simulink subsystem "PROGRAM_COUNTER_06_SS"  (R2022a)
settings: Solver=VariableStepAuto  StartTime=0.0  StopTime=10.0  RelTol=1e-3
libraries: hdlBasic x1928, hlsBasic x1
(part 1 of 12)
settings Model: Creator=sebas  LastModifiedBy=sebas

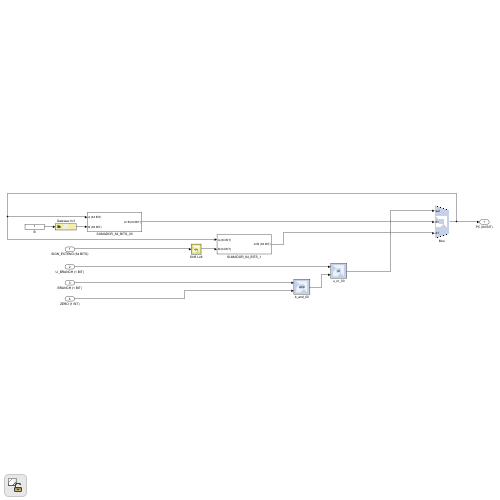
[thumbnail: Simulink's stored preview of the top-level diagram]
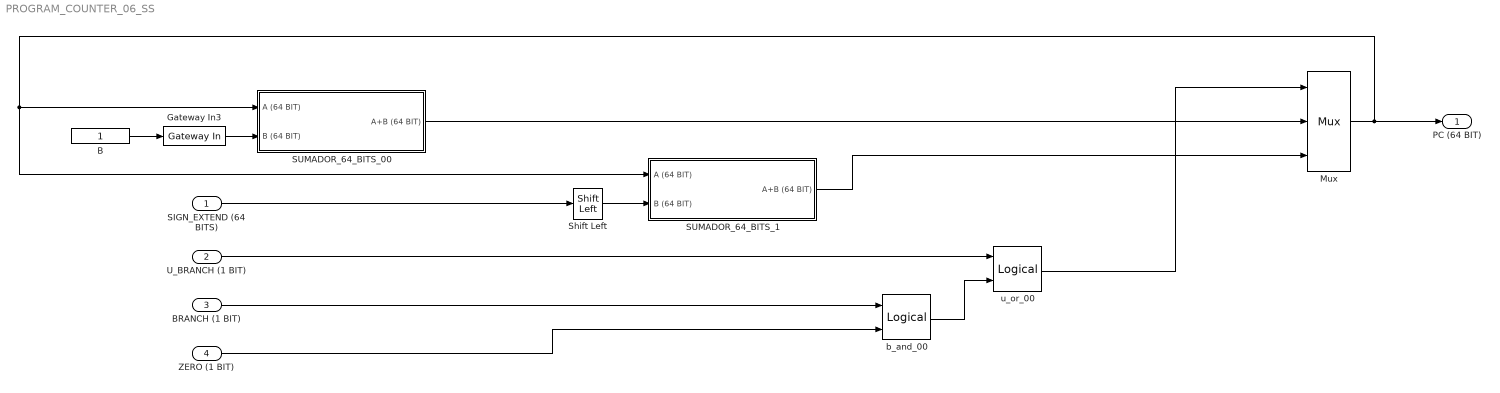
== system PROGRAM_COUNTER_06_SS ==
  SIGN_EXTEND (64 BITS) : Inport
  U_BRANCH (1 BIT) : Inport  Port=2
  BRANCH (1 BIT) : Inport  Port=3
  ZERO (1 BIT) : Inport  Port=4
  B : Constant
  Gateway In3 : hdlBasic/Gateway In  gui_display_data_type=Fixed-point  arith_type=Unsigned  n_bits=1  bin_pt=0  preci_type=Single  exp_width=8  frac_width=24  rows=1  columns=1  quantization="Round  (unbiased: +/- Inf)"  overflow=Saturate  period=1  UseAsADC=off  ADCChannel='1'  interface=None  automatic_assignment=on  address_offset=hex2dec('00')  intf_name=''  intf_description=''  default_value=0  timing_constraint=None  locs_specified=off  LOCs={}  io_standard={}  inherit_from_input=off  hdl_port=on  XmcBlockStatus=1  maskContainerNames=group4  block_type=gatewayin  block_config=sysgen:gateway_in_config  block_width_w=590  block_height_w=620  block_width=640  block_height=850
  Mux : hdlBasic/Mux  inputs=2  en=off  latency=0  precision=Full  arith_type=Unsigned  n_bits=16  bin_pt=14  quantization=Truncate  overflow=Wrap  XmcBlockStatus=1  maskContainerNames=tabcontainer1  block_type=mux  block_config=sysgen:Mux_config
  SUMADOR_64_BITS_00 : Subsystem
  SUMADOR_64_BITS_1 : Subsystem
  Shift Left : hlsBasic/Shift Left  ShiftAmount=2
  b_and_00 : hdlBasic/Logical  logical_function=AND  inputs=2  en=off  latency=0  precision=Full  arith_type=Unsigned  n_bits=16  bin_pt=0  align_bp=on  overflow=[]  quantization=[]  XmcBlockStatus=1  maskContainerNames=tabcontainer1  block_type=logical  block_config=sysgen:Logical_config
  u_or_00 : hdlBasic/Logical  logical_function=OR  inputs=2  en=off  latency=0  precision=Full  arith_type=Unsigned  n_bits=16  bin_pt=0  align_bp=on  overflow=[]  quantization=[]  XmcBlockStatus=1  maskContainerNames=tabcontainer1  block_type=logical  block_config=sysgen:Logical_config
  PC (64 BIT) : Outport
  wires:
  ZERO (1 BIT)/1 -> b_and_00/2
  SUMADOR_64_BITS_1/1(A+B (64 BIT)) -> Mux/3
  SUMADOR_64_BITS_00/1(A+B (64 BIT)) -> Mux/2
  u_or_00/1 -> Mux/1
  Gateway In3/1 -> SUMADOR_64_BITS_00/2(B (64 BIT))
  Mux/1 -> SUMADOR_64_BITS_00/1(A (64 BIT)), SUMADOR_64_BITS_1/1(A (64 BIT)), PC (64 BIT)/1
  BRANCH (1 BIT)/1 -> b_and_00/1
  B/1 -> Gateway In3/1
  U_BRANCH (1 BIT)/1 -> u_or_00/1
  SIGN_EXTEND (64 BITS)/1 -> Shift Left/1
  b_and_00/1 -> u_or_00/2
  Shift Left/1 -> SUMADOR_64_BITS_1/2(B (64 BIT))
